simulink model "VCU_CS75_12_27_test"  (R2014a)
settings: Solver=FixedStepDiscrete  StartTime=0.0  StopTime=25  FixedStep=0.0005  RelTol=1e-3
undefined symbols (not defined in the file): D1, D2, D3, ecucoder_acal, ErrorSumMax1, ErrorSumMax2, ErrorSumMax3, I1, I2, I3, I_SW01_L, LaterlAngleCommand, LDW, P1, P2, P3, RemoteAcclPosition
libraries: simulink x913, ec5744lib x39
(part 20 of 30)

== system VCU_CS75_12_27_test/长安CS75底盘程序，20ms一次/Output/Subsystem/TransmitMessages10/LAS_29D/LAS_VoiceWarning ==
  LAS_VoiceWarning : Inport
  Constant{1..2,4..8} (7 alike) : Constant  Value=0  OutDataTypeStr=uint8
  LAS_VoiceWarningRon : Rounding  Operator=round
  LAS_VoiceWarning_1sat : Saturate  UpperLimit=192  LowerLimit=0
  LAS_VoiceWarning_Convert : DataTypeConversion  OutDataTypeStr=uint8
  LAS_VoiceWarning_Convert1 : DataTypeConversion  OutDataTypeStr=uint32
  LAS_VoiceWarning_D : Product  Inputs=*/
  LAS_VoiceWarning_F : Constant  OutDataTypeStr=single
  LAS_VoiceWarning_L : simulink/Logic and Bit Operations/Bitwise Operator  logicop=AND  UseBitMask=on  BitMask=192  BitMaskRealWorld=Stored Integer
  LAS_VoiceWarning_O : Constant  Value=0  OutDataTypeStr=single
  LAS_VoiceWarning_S : ArithShift  BitShiftNumber=-6
  LAS_VoiceWarning_sat : Saturate  UpperLimit=0  LowerLimit=0
  LAS_VoiceWarning_st : Sum  Inputs=+-
  output1 : Outport
  output2 : Outport  Port=2
  output3 : Outport  Port=3
  output4 : Outport  Port=4
  output5 : Outport  Port=5
  output6 : Outport  Port=6
  output7 : Outport  Port=7
  output8 : Outport  Port=8
  wires:
  LAS_VoiceWarning/1 -> LAS_VoiceWarning_sat/1
  LAS_VoiceWarning_sat/1 -> LAS_VoiceWarning_st/1
  LAS_VoiceWarning_O/1 -> LAS_VoiceWarning_st/2
  LAS_VoiceWarning_st/1 -> LAS_VoiceWarning_D/1
  LAS_VoiceWarning_F/1 -> LAS_VoiceWarning_D/2
  LAS_VoiceWarning_D/1 -> LAS_VoiceWarningRon/1
  LAS_VoiceWarningRon/1 -> LAS_VoiceWarning_S/1
  LAS_VoiceWarning_S/1 -> LAS_VoiceWarning_1sat/1
  LAS_VoiceWarning_1sat/1 -> LAS_VoiceWarning_Convert1/1
  LAS_VoiceWarning_Convert1/1 -> LAS_VoiceWarning_L/1
  LAS_VoiceWarning_L/1 -> LAS_VoiceWarning_Convert/1
  LAS_VoiceWarning_Convert/1 -> output3/1
  Constant1/1 -> output1/1
  Constant2/1 -> output2/1
  Constant4/1 -> output4/1
  Constant5/1 -> output5/1
  Constant6/1 -> output6/1
  Constant7/1 -> output7/1
  Constant8/1 -> output8/1

== system VCU_CS75_12_27_test/长安CS75底盘程序，20ms一次/Output/Subsystem/TransmitMessages10/LAS_29D/RollingConter ==
  RollingConter : Inport
  Constant{1..6,8} (7 alike) : Constant  Value=0  OutDataTypeStr=uint8
  RollingConterRon : Rounding  Operator=round
  RollingConter_1sat : Saturate  UpperLimit=15  LowerLimit=0
  RollingConter_Convert : DataTypeConversion  OutDataTypeStr=uint8
  RollingConter_Convert1 : DataTypeConversion  OutDataTypeStr=uint32
  RollingConter_D : Product  Inputs=*/
  RollingConter_F : Constant  OutDataTypeStr=single
  RollingConter_L : simulink/Logic and Bit Operations/Bitwise Operator  logicop=AND  UseBitMask=on  BitMask=15  BitMaskRealWorld=Stored Integer
  RollingConter_O : Constant  Value=0  OutDataTypeStr=single
  RollingConter_S : ArithShift
  RollingConter_sat : Saturate  UpperLimit=0  LowerLimit=0
  RollingConter_st : Sum  Inputs=+-
  output1 : Outport
  output2 : Outport  Port=2
  output3 : Outport  Port=3
  output4 : Outport  Port=4
  output5 : Outport  Port=5
  output6 : Outport  Port=6
  output7 : Outport  Port=7
  output8 : Outport  Port=8
  wires:
  RollingConter/1 -> RollingConter_sat/1
  RollingConter_sat/1 -> RollingConter_st/1
  RollingConter_O/1 -> RollingConter_st/2
  RollingConter_st/1 -> RollingConter_D/1
  RollingConter_F/1 -> RollingConter_D/2
  RollingConter_D/1 -> RollingConterRon/1
  RollingConterRon/1 -> RollingConter_S/1
  RollingConter_S/1 -> RollingConter_1sat/1
  RollingConter_1sat/1 -> RollingConter_Convert1/1
  RollingConter_Convert1/1 -> RollingConter_L/1
  RollingConter_L/1 -> RollingConter_Convert/1
  RollingConter_Convert/1 -> output7/1
  Constant1/1 -> output1/1
  Constant2/1 -> output2/1
  Constant3/1 -> output3/1
  Constant4/1 -> output4/1
  Constant5/1 -> output5/1
  Constant6/1 -> output6/1
  Constant8/1 -> output8/1

== system VCU_CS75_12_27_test/长安CS75底盘程序，20ms一次/Output/Subsystem/TransmitMessages11/GW_LCDAL_2EA/LCDAL_AudioWarningEnableStatus ==
  LCDAL_AudioWarningEnableStatus : Inport
  Constant{1..4,6..8} (7 alike) : Constant  Value=0  OutDataTypeStr=uint8
  LCDAL_AudioWarningEnableStatusABS : Abs
  LCDAL_AudioWarningEnableStatusCS : ArithShift  BitShiftNumber=-2
  LCDAL_AudioWarningEnableStatusConS : Constant  OutDataTypeStr=single
  LCDAL_AudioWarningEnableStatusCosR : Constant  Value=0  OutDataTypeStr=uint8
  LCDAL_AudioWarningEnableStatusROP : RelationalOperator  Operator=<  OutDataTypeStr=boolean
  LCDAL_AudioWarningEnableStatusRon : Rounding  Operator=round
  LCDAL_AudioWarningEnableStatusSW : Switch  Criteria=u2 ~= 0
  LCDAL_AudioWarningEnableStatus_1sat : Saturate  UpperLimit=192  LowerLimit=0
  LCDAL_AudioWarningEnableStatus_Convert : DataTypeConversion  OutDataTypeStr=uint8
  LCDAL_AudioWarningEnableStatus_Convert1 : DataTypeConversion  OutDataTypeStr=uint32
  LCDAL_AudioWarningEnableStatus_D : Product  Inputs=*/
  LCDAL_AudioWarningEnableStatus_F : Constant  OutDataTypeStr=single
  LCDAL_AudioWarningEnableStatus_L : simulink/Logic and Bit Operations/Bitwise Operator  logicop=AND  UseBitMask=on  BitMask=192  BitMaskRealWorld=Stored Integer
  LCDAL_AudioWarningEnableStatus_O : Constant  Value=0  OutDataTypeStr=single
  LCDAL_AudioWarningEnableStatus_S : ArithShift  BitShiftNumber=-6
  LCDAL_AudioWarningEnableStatus_sat : Saturate  UpperLimit=3  LowerLimit=0
  LCDAL_AudioWarningEnableStatus_st : Sum  Inputs=+-
  LCDAL_AudioWarningEnableStatussubcon : Sum  Inputs=+-
  output1 : Outport
  output2 : Outport  Port=2
  output3 : Outport  Port=3
  output4 : Outport  Port=4
  output5 : Outport  Port=5
  output6 : Outport  Port=6
  output7 : Outport  Port=7
  output8 : Outport  Port=8
  wires:
  Constant8/1 -> output8/1
  Constant7/1 -> output7/1
  Constant6/1 -> output6/1
  Constant4/1 -> output4/1
  Constant3/1 -> output3/1
  Constant2/1 -> output2/1
  Constant1/1 -> output1/1
  LCDAL_AudioWarningEnableStatus_Convert/1 -> output5/1
  LCDAL_AudioWarningEnableStatus_L/1 -> LCDAL_AudioWarningEnableStatus_Convert/1
  LCDAL_AudioWarningEnableStatus_Convert1/1 -> LCDAL_AudioWarningEnableStatus_L/1
  LCDAL_AudioWarningEnableStatus_1sat/1 -> LCDAL_AudioWarningEnableStatus_Convert1/1
  LCDAL_AudioWarningEnableStatus_S/1 -> LCDAL_AudioWarningEnableStatus_1sat/1
  LCDAL_AudioWarningEnableStatusSW/1 -> LCDAL_AudioWarningEnableStatus_S/1
  LCDAL_AudioWarningEnableStatusROP/1 -> LCDAL_AudioWarningEnableStatusSW/2
  LCDAL_AudioWarningEnableStatussubcon/1 -> LCDAL_AudioWarningEnableStatusSW/1
  LCDAL_AudioWarningEnableStatusABS/1 -> LCDAL_AudioWarningEnableStatussubcon/2
  LCDAL_AudioWarningEnableStatusCS/1 -> LCDAL_AudioWarningEnableStatussubcon/1
  LCDAL_AudioWarningEnableStatusConS/1 -> LCDAL_AudioWarningEnableStatusCS/1
  LCDAL_AudioWarningEnableStatusCosR/1 -> LCDAL_AudioWarningEnableStatusROP/2
  LCDAL_AudioWarningEnableStatusRon/1 -> LCDAL_AudioWarningEnableStatusSW/3, LCDAL_AudioWarningEnableStatusABS/1, LCDAL_AudioWarningEnableStatusROP/1
  LCDAL_AudioWarningEnableStatus_D/1 -> LCDAL_AudioWarningEnableStatusRon/1
  LCDAL_AudioWarningEnableStatus_F/1 -> LCDAL_AudioWarningEnableStatus_D/2
  LCDAL_AudioWarningEnableStatus_st/1 -> LCDAL_AudioWarningEnableStatus_D/1
  LCDAL_AudioWarningEnableStatus_O/1 -> LCDAL_AudioWarningEnableStatus_st/2
  LCDAL_AudioWarningEnableStatus_sat/1 -> LCDAL_AudioWarningEnableStatus_st/1
  LCDAL_AudioWarningEnableStatus/1 -> LCDAL_AudioWarningEnableStatus_sat/1

== system VCU_CS75_12_27_test/长安CS75底盘程序，20ms一次/Output/Subsystem/TransmitMessages11/GW_LCDAL_2EA/LCDAL_BSDLCAAlert ==
  LCDAL_BSDLCAAlert : Inport
  Constant{2..8} (7 alike) : Constant  Value=0  OutDataTypeStr=uint8
  LCDAL_BSDLCAAlertRon : Rounding  Operator=round
  LCDAL_BSDLCAAlert_1sat : Saturate  UpperLimit=48  LowerLimit=0
  LCDAL_BSDLCAAlert_Convert : DataTypeConversion  OutDataTypeStr=uint8
  LCDAL_BSDLCAAlert_Convert1 : DataTypeConversion  OutDataTypeStr=uint32
  LCDAL_BSDLCAAlert_D : Product  Inputs=*/
  LCDAL_BSDLCAAlert_F : Constant  OutDataTypeStr=single
  LCDAL_BSDLCAAlert_L : simulink/Logic and Bit Operations/Bitwise Operator  logicop=AND  UseBitMask=on  BitMask=48  BitMaskRealWorld=Stored Integer
  LCDAL_BSDLCAAlert_O : Constant  Value=0  OutDataTypeStr=single
  LCDAL_BSDLCAAlert_S : ArithShift  BitShiftNumber=-4
  LCDAL_BSDLCAAlert_sat : Saturate  UpperLimit=3  LowerLimit=0
  LCDAL_BSDLCAAlert_st : Sum  Inputs=+-
  output1 : Outport
  output2 : Outport  Port=2
  output3 : Outport  Port=3
  output4 : Outport  Port=4
  output5 : Outport  Port=5
  output6 : Outport  Port=6
  output7 : Outport  Port=7
  output8 : Outport  Port=8
  wires:
  Constant8/1 -> output8/1
  Constant7/1 -> output7/1
  Constant6/1 -> output6/1
  Constant5/1 -> output5/1
  Constant4/1 -> output4/1
  Constant3/1 -> output3/1
  Constant2/1 -> output2/1
  LCDAL_BSDLCAAlert_Convert/1 -> output1/1
  LCDAL_BSDLCAAlert_L/1 -> LCDAL_BSDLCAAlert_Convert/1
  LCDAL_BSDLCAAlert_Convert1/1 -> LCDAL_BSDLCAAlert_L/1
  LCDAL_BSDLCAAlert_1sat/1 -> LCDAL_BSDLCAAlert_Convert1/1
  LCDAL_BSDLCAAlert_S/1 -> LCDAL_BSDLCAAlert_1sat/1
  LCDAL_BSDLCAAlertRon/1 -> LCDAL_BSDLCAAlert_S/1
  LCDAL_BSDLCAAlert_D/1 -> LCDAL_BSDLCAAlertRon/1
  LCDAL_BSDLCAAlert_F/1 -> LCDAL_BSDLCAAlert_D/2
  LCDAL_BSDLCAAlert_st/1 -> LCDAL_BSDLCAAlert_D/1
  LCDAL_BSDLCAAlert_O/1 -> LCDAL_BSDLCAAlert_st/2
  LCDAL_BSDLCAAlert_sat/1 -> LCDAL_BSDLCAAlert_st/1
  LCDAL_BSDLCAAlert/1 -> LCDAL_BSDLCAAlert_sat/1

== system VCU_CS75_12_27_test/长安CS75底盘程序，20ms一次/Output/Subsystem/TransmitMessages11/GW_LCDAL_2EA/LCDAL_BSDLCAEnableStatus ==
  LCDAL_BSDLCAEnableStatus : Inport
  Constant{2..8} (7 alike) : Constant  Value=0  OutDataTypeStr=uint8
  LCDAL_BSDLCAEnableStatusRon : Rounding  Operator=round
  LCDAL_BSDLCAEnableStatus_1sat : Saturate  UpperLimit=192  LowerLimit=0
  LCDAL_BSDLCAEnableStatus_Convert : DataTypeConversion  OutDataTypeStr=uint8
  LCDAL_BSDLCAEnableStatus_Convert1 : DataTypeConversion  OutDataTypeStr=uint32
  LCDAL_BSDLCAEnableStatus_D : Product  Inputs=*/
  LCDAL_BSDLCAEnableStatus_F : Constant  OutDataTypeStr=single
  LCDAL_BSDLCAEnableStatus_L : simulink/Logic and Bit Operations/Bitwise Operator  logicop=AND  UseBitMask=on  BitMask=192  BitMaskRealWorld=Stored Integer
  LCDAL_BSDLCAEnableStatus_O : Constant  Value=0  OutDataTypeStr=single
  LCDAL_BSDLCAEnableStatus_S : ArithShift  BitShiftNumber=-6
  LCDAL_BSDLCAEnableStatus_sat : Saturate  UpperLimit=3  LowerLimit=0
  LCDAL_BSDLCAEnableStatus_st : Sum  Inputs=+-
  output1 : Outport
  output2 : Outport  Port=2
  output3 : Outport  Port=3
  output4 : Outport  Port=4
  output5 : Outport  Port=5
  output6 : Outport  Port=6
  output7 : Outport  Port=7
  output8 : Outport  Port=8
  wires:
  Constant8/1 -> output8/1
  Constant7/1 -> output7/1
  Constant6/1 -> output6/1
  Constant5/1 -> output5/1
  Constant4/1 -> output4/1
  Constant3/1 -> output3/1
  Constant2/1 -> output2/1
  LCDAL_BSDLCAEnableStatus_Convert/1 -> output1/1
  LCDAL_BSDLCAEnableStatus_L/1 -> LCDAL_BSDLCAEnableStatus_Convert/1
  LCDAL_BSDLCAEnableStatus_Convert1/1 -> LCDAL_BSDLCAEnableStatus_L/1
  LCDAL_BSDLCAEnableStatus_1sat/1 -> LCDAL_BSDLCAEnableStatus_Convert1/1
  LCDAL_BSDLCAEnableStatus_S/1 -> LCDAL_BSDLCAEnableStatus_1sat/1
  LCDAL_BSDLCAEnableStatusRon/1 -> LCDAL_BSDLCAEnableStatus_S/1
  LCDAL_BSDLCAEnableStatus_D/1 -> LCDAL_BSDLCAEnableStatusRon/1
  LCDAL_BSDLCAEnableStatus_F/1 -> LCDAL_BSDLCAEnableStatus_D/2
  LCDAL_BSDLCAEnableStatus_st/1 -> LCDAL_BSDLCAEnableStatus_D/1
  LCDAL_BSDLCAEnableStatus_O/1 -> LCDAL_BSDLCAEnableStatus_st/2
  LCDAL_BSDLCAEnableStatus_sat/1 -> LCDAL_BSDLCAEnableStatus_st/1
  LCDAL_BSDLCAEnableStatus/1 -> LCDAL_BSDLCAEnableStatus_sat/1

== system VCU_CS75_12_27_test/长安CS75底盘程序，20ms一次/Output/Subsystem/TransmitMessages11/GW_LCDAL_2EA/LCDAL_BSDLCAStatus ==
  LCDAL_BSDLCAStatus : Inport
  Constant{1,3..8} (7 alike) : Constant  Value=0  OutDataTypeStr=uint8
  LCDAL_BSDLCAStatusRon : Rounding  Operator=round
  LCDAL_BSDLCAStatus_1sat : Saturate  UpperLimit=24  LowerLimit=0
  LCDAL_BSDLCAStatus_Convert : DataTypeConversion  OutDataTypeStr=uint8
  LCDAL_BSDLCAStatus_Convert1 : DataTypeConversion  OutDataTypeStr=uint32
  LCDAL_BSDLCAStatus_D : Product  Inputs=*/
  LCDAL_BSDLCAStatus_F : Constant  OutDataTypeStr=single
  LCDAL_BSDLCAStatus_L : simulink/Logic and Bit Operations/Bitwise Operator  logicop=AND  UseBitMask=on  BitMask=24  BitMaskRealWorld=Stored Integer
  LCDAL_BSDLCAStatus_O : Constant  Value=0  OutDataTypeStr=single
  LCDAL_BSDLCAStatus_S : ArithShift  BitShiftNumber=-3
  LCDAL_BSDLCAStatus_sat : Saturate  UpperLimit=3  LowerLimit=0
  LCDAL_BSDLCAStatus_st : Sum  Inputs=+-
  output1 : Outport
  output2 : Outport  Port=2
  output3 : Outport  Port=3
  output4 : Outport  Port=4
  output5 : Outport  Port=5
  output6 : Outport  Port=6
  output7 : Outport  Port=7
  output8 : Outport  Port=8
  wires:
  Constant8/1 -> output8/1
  Constant7/1 -> output7/1
  Constant6/1 -> output6/1
  Constant5/1 -> output5/1
  Constant4/1 -> output4/1
  Constant3/1 -> output3/1
  Constant1/1 -> output1/1
  LCDAL_BSDLCAStatus_Convert/1 -> output2/1
  LCDAL_BSDLCAStatus_L/1 -> LCDAL_BSDLCAStatus_Convert/1
  LCDAL_BSDLCAStatus_Convert1/1 -> LCDAL_BSDLCAStatus_L/1
  LCDAL_BSDLCAStatus_1sat/1 -> LCDAL_BSDLCAStatus_Convert1/1
  LCDAL_BSDLCAStatus_S/1 -> LCDAL_BSDLCAStatus_1sat/1
  LCDAL_BSDLCAStatusRon/1 -> LCDAL_BSDLCAStatus_S/1
  LCDAL_BSDLCAStatus_D/1 -> LCDAL_BSDLCAStatusRon/1
  LCDAL_BSDLCAStatus_F/1 -> LCDAL_BSDLCAStatus_D/2
  LCDAL_BSDLCAStatus_st/1 -> LCDAL_BSDLCAStatus_D/1
  LCDAL_BSDLCAStatus_O/1 -> LCDAL_BSDLCAStatus_st/2
  LCDAL_BSDLCAStatus_sat/1 -> LCDAL_BSDLCAStatus_st/1
  LCDAL_BSDLCAStatus/1 -> LCDAL_BSDLCAStatus_sat/1

== system VCU_CS75_12_27_test/长安CS75底盘程序，20ms一次/Output/Subsystem/TransmitMessages11/GW_LCDAL_2EA/LCDAL_CTAAlert ==
  LCDAL_CTAAlert : Inport
  Constant{2..8} (7 alike) : Constant  Value=0  OutDataTypeStr=uint8
  LCDAL_CTAAlertABS : Abs
  LCDAL_CTAAlertCS : ArithShift  BitShiftNumber=-2
  LCDAL_CTAAlertConS : Constant  OutDataTypeStr=single
  LCDAL_CTAAlertCosR : Constant  Value=0  OutDataTypeStr=uint8
  LCDAL_CTAAlertROP : RelationalOperator  Operator=<  OutDataTypeStr=boolean
  LCDAL_CTAAlertRon : Rounding  Operator=round
  LCDAL_CTAAlertSW : Switch  Criteria=u2 ~= 0
  LCDAL_CTAAlert_1sat : Saturate  UpperLimit=3  LowerLimit=0
  LCDAL_CTAAlert_Convert : DataTypeConversion  OutDataTypeStr=uint8
  LCDAL_CTAAlert_Convert1 : DataTypeConversion  OutDataTypeStr=uint32
  LCDAL_CTAAlert_D : Product  Inputs=*/
  LCDAL_CTAAlert_F : Constant  OutDataTypeStr=single
  LCDAL_CTAAlert_L : simulink/Logic and Bit Operations/Bitwise Operator  logicop=AND  UseBitMask=on  BitMask=3  BitMaskRealWorld=Stored Integer
  LCDAL_CTAAlert_O : Constant  Value=0  OutDataTypeStr=single
  LCDAL_CTAAlert_S : ArithShift
  LCDAL_CTAAlert_sat : Saturate  UpperLimit=3  LowerLimit=0
  LCDAL_CTAAlert_st : Sum  Inputs=+-
  LCDAL_CTAAlertsubcon : Sum  Inputs=+-
  output1 : Outport
  output2 : Outport  Port=2
  output3 : Outport  Port=3
  output4 : Outport  Port=4
  output5 : Outport  Port=5
  output6 : Outport  Port=6
  output7 : Outport  Port=7
  output8 : Outport  Port=8
  wires:
  Constant8/1 -> output8/1
  Constant7/1 -> output7/1
  Constant6/1 -> output6/1
  Constant5/1 -> output5/1
  Constant4/1 -> output4/1
  Constant3/1 -> output3/1
  Constant2/1 -> output2/1
  LCDAL_CTAAlert_Convert/1 -> output1/1
  LCDAL_CTAAlert_L/1 -> LCDAL_CTAAlert_Convert/1
  LCDAL_CTAAlert_Convert1/1 -> LCDAL_CTAAlert_L/1
  LCDAL_CTAAlert_1sat/1 -> LCDAL_CTAAlert_Convert1/1
  LCDAL_CTAAlert_S/1 -> LCDAL_CTAAlert_1sat/1
  LCDAL_CTAAlertSW/1 -> LCDAL_CTAAlert_S/1
  LCDAL_CTAAlertROP/1 -> LCDAL_CTAAlertSW/2
  LCDAL_CTAAlertsubcon/1 -> LCDAL_CTAAlertSW/1
  LCDAL_CTAAlertABS/1 -> LCDAL_CTAAlertsubcon/2
  LCDAL_CTAAlertCS/1 -> LCDAL_CTAAlertsubcon/1
  LCDAL_CTAAlertConS/1 -> LCDAL_CTAAlertCS/1
  LCDAL_CTAAlertCosR/1 -> LCDAL_CTAAlertROP/2
  LCDAL_CTAAlertRon/1 -> LCDAL_CTAAlertSW/3, LCDAL_CTAAlertABS/1, LCDAL_CTAAlertROP/1
  LCDAL_CTAAlert_D/1 -> LCDAL_CTAAlertRon/1
  LCDAL_CTAAlert_F/1 -> LCDAL_CTAAlert_D/2
  LCDAL_CTAAlert_st/1 -> LCDAL_CTAAlert_D/1
  LCDAL_CTAAlert_O/1 -> LCDAL_CTAAlert_st/2
  LCDAL_CTAAlert_sat/1 -> LCDAL_CTAAlert_st/1
  LCDAL_CTAAlert/1 -> LCDAL_CTAAlert_sat/1

== system VCU_CS75_12_27_test/长安CS75底盘程序，20ms一次/Output/Subsystem/TransmitMessages11/GW_LCDAL_2EA/LCDAL_CTAEnableStatus ==
  LCDAL_CTAEnableStatus : Inport
  Constant{1..3,5..8} (7 alike) : Constant  Value=0  OutDataTypeStr=uint8
  LCDAL_CTAEnableStatusRon : Rounding  Operator=round
  LCDAL_CTAEnableStatus_1sat : Saturate  UpperLimit=192  LowerLimit=0
  LCDAL_CTAEnableStatus_Convert : DataTypeConversion  OutDataTypeStr=uint8
  LCDAL_CTAEnableStatus_Convert1 : DataTypeConversion  OutDataTypeStr=uint32
  LCDAL_CTAEnableStatus_D : Product  Inputs=*/
  LCDAL_CTAEnableStatus_F : Constant  OutDataTypeStr=single
  LCDAL_CTAEnableStatus_L : simulink/Logic and Bit Operations/Bitwise Operator  logicop=AND  UseBitMask=on  BitMask=192  BitMaskRealWorld=Stored Integer
  LCDAL_CTAEnableStatus_O : Constant  Value=0  OutDataTypeStr=single
  LCDAL_CTAEnableStatus_S : ArithShift  BitShiftNumber=-6
  LCDAL_CTAEnableStatus_sat : Saturate  UpperLimit=3  LowerLimit=0
  LCDAL_CTAEnableStatus_st : Sum  Inputs=+-
  output1 : Outport
  output2 : Outport  Port=2
  output3 : Outport  Port=3
  output4 : Outport  Port=4
  output5 : Outport  Port=5
  output6 : Outport  Port=6
  output7 : Outport  Port=7
  output8 : Outport  Port=8
  wires:
  Constant8/1 -> output8/1
  Constant7/1 -> output7/1
  Constant6/1 -> output6/1
  Constant5/1 -> output5/1
  Constant3/1 -> output3/1
  Constant2/1 -> output2/1
  Constant1/1 -> output1/1
  LCDAL_CTAEnableStatus_Convert/1 -> output4/1
  LCDAL_CTAEnableStatus_L/1 -> LCDAL_CTAEnableStatus_Convert/1
  LCDAL_CTAEnableStatus_Convert1/1 -> LCDAL_CTAEnableStatus_L/1
  LCDAL_CTAEnableStatus_1sat/1 -> LCDAL_CTAEnableStatus_Convert1/1
  LCDAL_CTAEnableStatus_S/1 -> LCDAL_CTAEnableStatus_1sat/1
  LCDAL_CTAEnableStatusRon/1 -> LCDAL_CTAEnableStatus_S/1
  LCDAL_CTAEnableStatus_D/1 -> LCDAL_CTAEnableStatusRon/1
  LCDAL_CTAEnableStatus_F/1 -> LCDAL_CTAEnableStatus_D/2
  LCDAL_CTAEnableStatus_st/1 -> LCDAL_CTAEnableStatus_D/1
  LCDAL_CTAEnableStatus_O/1 -> LCDAL_CTAEnableStatus_st/2
  LCDAL_CTAEnableStatus_sat/1 -> LCDAL_CTAEnableStatus_st/1
  LCDAL_CTAEnableStatus/1 -> LCDAL_CTAEnableStatus_sat/1

== system VCU_CS75_12_27_test/长安CS75底盘程序，20ms一次/Output/Subsystem/TransmitMessages11/GW_LCDAL_2EA/LCDAL_CTAStatus ==
  LCDAL_CTAStatus : Inport
  Constant{1,3..8} (7 alike) : Constant  Value=0  OutDataTypeStr=uint8
  LCDAL_CTAStatusRon : Rounding  Operator=round
  LCDAL_CTAStatus_1sat : Saturate  UpperLimit=6  LowerLimit=0
  LCDAL_CTAStatus_Convert : DataTypeConversion  OutDataTypeStr=uint8
  LCDAL_CTAStatus_Convert1 : DataTypeConversion  OutDataTypeStr=uint32
  LCDAL_CTAStatus_D : Product  Inputs=*/
  LCDAL_CTAStatus_F : Constant  OutDataTypeStr=single
  LCDAL_CTAStatus_L : simulink/Logic and Bit Operations/Bitwise Operator  logicop=AND  UseBitMask=on  BitMask=6  BitMaskRealWorld=Stored Integer
  LCDAL_CTAStatus_O : Constant  Value=0  OutDataTypeStr=single
  LCDAL_CTAStatus_S : ArithShift  BitShiftNumber=-1
  LCDAL_CTAStatus_sat : Saturate  UpperLimit=3  LowerLimit=0
  LCDAL_CTAStatus_st : Sum  Inputs=+-
  output1 : Outport
  output2 : Outport  Port=2
  output3 : Outport  Port=3
  output4 : Outport  Port=4
  output5 : Outport  Port=5
  output6 : Outport  Port=6
  output7 : Outport  Port=7
  output8 : Outport  Port=8
  wires:
  Constant8/1 -> output8/1
  Constant7/1 -> output7/1
  Constant6/1 -> output6/1
  Constant5/1 -> output5/1
  Constant4/1 -> output4/1
  Constant3/1 -> output3/1
  Constant1/1 -> output1/1
  LCDAL_CTAStatus_Convert/1 -> output2/1
  LCDAL_CTAStatus_L/1 -> LCDAL_CTAStatus_Convert/1
  LCDAL_CTAStatus_Convert1/1 -> LCDAL_CTAStatus_L/1
  LCDAL_CTAStatus_1sat/1 -> LCDAL_CTAStatus_Convert1/1
  LCDAL_CTAStatus_S/1 -> LCDAL_CTAStatus_1sat/1
  LCDAL_CTAStatusRon/1 -> LCDAL_CTAStatus_S/1
  LCDAL_CTAStatus_D/1 -> LCDAL_CTAStatusRon/1
  LCDAL_CTAStatus_F/1 -> LCDAL_CTAStatus_D/2
  LCDAL_CTAStatus_st/1 -> LCDAL_CTAStatus_D/1
  LCDAL_CTAStatus_O/1 -> LCDAL_CTAStatus_st/2
  LCDAL_CTAStatus_sat/1 -> LCDAL_CTAStatus_st/1
  LCDAL_CTAStatus/1 -> LCDAL_CTAStatus_sat/1

== system VCU_CS75_12_27_test/长安CS75底盘程序，20ms一次/Output/Subsystem/TransmitMessages11/GW_LCDAL_2EA/LCDAL_LCATTCSettingStatus ==
  LCDAL_LCATTCSettingStatus : Inport
  Constant{1..4,6..8} (7 alike) : Constant  Value=0  OutDataTypeStr=uint8
  LCDAL_LCATTCSettingStatusABS : Abs
  LCDAL_LCATTCSettingStatusCS : ArithShift  BitShiftNumber=-2
  LCDAL_LCATTCSettingStatusConS : Constant  OutDataTypeStr=single
  LCDAL_LCATTCSettingStatusCosR : Constant  Value=0  OutDataTypeStr=uint8
  LCDAL_LCATTCSettingStatusROP : RelationalOperator  Operator=<  OutDataTypeStr=boolean
  LCDAL_LCATTCSettingStatusRon : Rounding  Operator=round
  LCDAL_LCATTCSettingStatusSW : Switch  Criteria=u2 ~= 0
  LCDAL_LCATTCSettingStatus_1sat : Saturate  UpperLimit=12  LowerLimit=0
  LCDAL_LCATTCSettingStatus_Convert : DataTypeConversion  OutDataTypeStr=uint8
  LCDAL_LCATTCSettingStatus_Convert1 : DataTypeConversion  OutDataTypeStr=uint32
  LCDAL_LCATTCSettingStatus_D : Product  Inputs=*/
  LCDAL_LCATTCSettingStatus_F : Constant  OutDataTypeStr=single
  LCDAL_LCATTCSettingStatus_L : simulink/Logic and Bit Operations/Bitwise Operator  logicop=AND  UseBitMask=on  BitMask=12  BitMaskRealWorld=Stored Integer
  LCDAL_LCATTCSettingStatus_O : Constant  Value=0  OutDataTypeStr=single
  LCDAL_LCATTCSettingStatus_S : ArithShift  BitShiftNumber=-2
  LCDAL_LCATTCSettingStatus_sat : Saturate  UpperLimit=3  LowerLimit=0
  LCDAL_LCATTCSettingStatus_st : Sum  Inputs=+-
  LCDAL_LCATTCSettingStatussubcon : Sum  Inputs=+-
  output1 : Outport
  output2 : Outport  Port=2
  output3 : Outport  Port=3
  output4 : Outport  Port=4
  output5 : Outport  Port=5
  output6 : Outport  Port=6
  output7 : Outport  Port=7
  output8 : Outport  Port=8
  wires:
  Constant8/1 -> output8/1
  Constant7/1 -> output7/1
  Constant6/1 -> output6/1
  Constant4/1 -> output4/1
  Constant3/1 -> output3/1
  Constant2/1 -> output2/1
  Constant1/1 -> output1/1
  LCDAL_LCATTCSettingStatus_Convert/1 -> output5/1
  LCDAL_LCATTCSettingStatus_L/1 -> LCDAL_LCATTCSettingStatus_Convert/1
  LCDAL_LCATTCSettingStatus_Convert1/1 -> LCDAL_LCATTCSettingStatus_L/1
  LCDAL_LCATTCSettingStatus_1sat/1 -> LCDAL_LCATTCSettingStatus_Convert1/1
  LCDAL_LCATTCSettingStatus_S/1 -> LCDAL_LCATTCSettingStatus_1sat/1
  LCDAL_LCATTCSettingStatusSW/1 -> LCDAL_LCATTCSettingStatus_S/1
  LCDAL_LCATTCSettingStatusROP/1 -> LCDAL_LCATTCSettingStatusSW/2
  LCDAL_LCATTCSettingStatussubcon/1 -> LCDAL_LCATTCSettingStatusSW/1
  LCDAL_LCATTCSettingStatusABS/1 -> LCDAL_LCATTCSettingStatussubcon/2
  LCDAL_LCATTCSettingStatusCS/1 -> LCDAL_LCATTCSettingStatussubcon/1
  LCDAL_LCATTCSettingStatusConS/1 -> LCDAL_LCATTCSettingStatusCS/1
  LCDAL_LCATTCSettingStatusCosR/1 -> LCDAL_LCATTCSettingStatusROP/2
  LCDAL_LCATTCSettingStatusRon/1 -> LCDAL_LCATTCSettingStatusSW/3, LCDAL_LCATTCSettingStatusABS/1, LCDAL_LCATTCSettingStatusROP/1
  LCDAL_LCATTCSettingStatus_D/1 -> LCDAL_LCATTCSettingStatusRon/1
  LCDAL_LCATTCSettingStatus_F/1 -> LCDAL_LCATTCSettingStatus_D/2
  LCDAL_LCATTCSettingStatus_st/1 -> LCDAL_LCATTCSettingStatus_D/1
  LCDAL_LCATTCSettingStatus_O/1 -> LCDAL_LCATTCSettingStatus_st/2
  LCDAL_LCATTCSettingStatus_sat/1 -> LCDAL_LCATTCSettingStatus_st/1
  LCDAL_LCATTCSettingStatus/1 -> LCDAL_LCATTCSettingStatus_sat/1

== system VCU_CS75_12_27_test/长安CS75底盘程序，20ms一次/Output/Subsystem/TransmitMessages11/GW_LCDAL_2EA/LCDAL_LockCtrlEnableStatus ==
  LCDAL_LockCtrlEnableStatus : Inport
  Constant{1..4,6..8} (7 alike) : Constant  Value=0  OutDataTypeStr=uint8
  LCDAL_LockCtrlEnableStatusABS : Abs
  LCDAL_LockCtrlEnableStatusCS : ArithShift  BitShiftNumber=-2
  LCDAL_LockCtrlEnableStatusConS : Constant  OutDataTypeStr=single
  LCDAL_LockCtrlEnableStatusCosR : Constant  Value=0  OutDataTypeStr=uint8
  LCDAL_LockCtrlEnableStatusROP : RelationalOperator  Operator=<  OutDataTypeStr=boolean
  LCDAL_LockCtrlEnableStatusRon : Rounding  Operator=round
  LCDAL_LockCtrlEnableStatusSW : Switch  Criteria=u2 ~= 0
  LCDAL_LockCtrlEnableStatus_1sat : Saturate  UpperLimit=48  LowerLimit=0
  LCDAL_LockCtrlEnableStatus_Convert : DataTypeConversion  OutDataTypeStr=uint8
  LCDAL_LockCtrlEnableStatus_Convert1 : DataTypeConversion  OutDataTypeStr=uint32
  LCDAL_LockCtrlEnableStatus_D : Product  Inputs=*/
  LCDAL_LockCtrlEnableStatus_F : Constant  OutDataTypeStr=single
  LCDAL_LockCtrlEnableStatus_L : simulink/Logic and Bit Operations/Bitwise Operator  logicop=AND  UseBitMask=on  BitMask=48  BitMaskRealWorld=Stored Integer
  LCDAL_LockCtrlEnableStatus_O : Constant  Value=0  OutDataTypeStr=single
  LCDAL_LockCtrlEnableStatus_S : ArithShift  BitShiftNumber=-4
  LCDAL_LockCtrlEnableStatus_sat : Saturate  UpperLimit=3  LowerLimit=0
  LCDAL_LockCtrlEnableStatus_st : Sum  Inputs=+-
  LCDAL_LockCtrlEnableStatussubcon : Sum  Inputs=+-
  output1 : Outport
  output2 : Outport  Port=2
  output3 : Outport  Port=3
  output4 : Outport  Port=4
  output5 : Outport  Port=5
  output6 : Outport  Port=6
  output7 : Outport  Port=7
  output8 : Outport  Port=8
  wires:
  Constant8/1 -> output8/1
  Constant7/1 -> output7/1
  Constant6/1 -> output6/1
  Constant4/1 -> output4/1
  Constant3/1 -> output3/1
  Constant2/1 -> output2/1
  Constant1/1 -> output1/1
  LCDAL_LockCtrlEnableStatus_Convert/1 -> output5/1
  LCDAL_LockCtrlEnableStatus_L/1 -> LCDAL_LockCtrlEnableStatus_Convert/1
  LCDAL_LockCtrlEnableStatus_Convert1/1 -> LCDAL_LockCtrlEnableStatus_L/1
  LCDAL_LockCtrlEnableStatus_1sat/1 -> LCDAL_LockCtrlEnableStatus_Convert1/1
  LCDAL_LockCtrlEnableStatus_S/1 -> LCDAL_LockCtrlEnableStatus_1sat/1
  LCDAL_LockCtrlEnableStatusSW/1 -> LCDAL_LockCtrlEnableStatus_S/1
  LCDAL_LockCtrlEnableStatusROP/1 -> LCDAL_LockCtrlEnableStatusSW/2
  LCDAL_LockCtrlEnableStatussubcon/1 -> LCDAL_LockCtrlEnableStatusSW/1
  LCDAL_LockCtrlEnableStatusABS/1 -> LCDAL_LockCtrlEnableStatussubcon/2
  LCDAL_LockCtrlEnableStatusCS/1 -> LCDAL_LockCtrlEnableStatussubcon/1
  LCDAL_LockCtrlEnableStatusConS/1 -> LCDAL_LockCtrlEnableStatusCS/1
  LCDAL_LockCtrlEnableStatusCosR/1 -> LCDAL_LockCtrlEnableStatusROP/2
  LCDAL_LockCtrlEnableStatusRon/1 -> LCDAL_LockCtrlEnableStatusSW/3, LCDAL_LockCtrlEnableStatusABS/1, LCDAL_LockCtrlEnableStatusROP/1
  LCDAL_LockCtrlEnableStatus_D/1 -> LCDAL_LockCtrlEnableStatusRon/1
  LCDAL_LockCtrlEnableStatus_F/1 -> LCDAL_LockCtrlEnableStatus_D/2
  LCDAL_LockCtrlEnableStatus_st/1 -> LCDAL_LockCtrlEnableStatus_D/1
  LCDAL_LockCtrlEnableStatus_O/1 -> LCDAL_LockCtrlEnableStatus_st/2
  LCDAL_LockCtrlEnableStatus_sat/1 -> LCDAL_LockCtrlEnableStatus_st/1
  LCDAL_LockCtrlEnableStatus/1 -> LCDAL_LockCtrlEnableStatus_sat/1

== system VCU_CS75_12_27_test/长安CS75底盘程序，20ms一次/Output/Subsystem/TransmitMessages11/GW_LCDAL_2EA/LCDAL_RCWAlert ==
  LCDAL_RCWAlert : Inport
  Constant{1..2,4..8} (7 alike) : Constant  Value=0  OutDataTypeStr=uint8
  LCDAL_RCWAlertRon : Rounding  Operator=round
  LCDAL_RCWAlert_1sat : Saturate  UpperLimit=3  LowerLimit=0
  LCDAL_RCWAlert_Convert : DataTypeConversion  OutDataTypeStr=uint8
  LCDAL_RCWAlert_Convert1 : DataTypeConversion  OutDataTypeStr=uint32
  LCDAL_RCWAlert_D : Product  Inputs=*/
  LCDAL_RCWAlert_F : Constant  OutDataTypeStr=single
  LCDAL_RCWAlert_L : simulink/Logic and Bit Operations/Bitwise Operator  logicop=AND  UseBitMask=on  BitMask=3  BitMaskRealWorld=Stored Integer
  LCDAL_RCWAlert_O : Constant  Value=0  OutDataTypeStr=single
  LCDAL_RCWAlert_S : ArithShift
  LCDAL_RCWAlert_sat : Saturate  UpperLimit=3  LowerLimit=0
  LCDAL_RCWAlert_st : Sum  Inputs=+-
  output1 : Outport
  output2 : Outport  Port=2
  output3 : Outport  Port=3
  output4 : Outport  Port=4
  output5 : Outport  Port=5
  output6 : Outport  Port=6
  output7 : Outport  Port=7
  output8 : Outport  Port=8
  wires:
  Constant8/1 -> output8/1
  Constant7/1 -> output7/1
  Constant6/1 -> output6/1
  Constant5/1 -> output5/1
  Constant4/1 -> output4/1
  Constant2/1 -> output2/1
  Constant1/1 -> output1/1
  LCDAL_RCWAlert_Convert/1 -> output3/1
  LCDAL_RCWAlert_L/1 -> LCDAL_RCWAlert_Convert/1
  LCDAL_RCWAlert_Convert1/1 -> LCDAL_RCWAlert_L/1
  LCDAL_RCWAlert_1sat/1 -> LCDAL_RCWAlert_Convert1/1
  LCDAL_RCWAlert_S/1 -> LCDAL_RCWAlert_1sat/1
  LCDAL_RCWAlertRon/1 -> LCDAL_RCWAlert_S/1
  LCDAL_RCWAlert_D/1 -> LCDAL_RCWAlertRon/1
  LCDAL_RCWAlert_F/1 -> LCDAL_RCWAlert_D/2
  LCDAL_RCWAlert_st/1 -> LCDAL_RCWAlert_D/1
  LCDAL_RCWAlert_O/1 -> LCDAL_RCWAlert_st/2
  LCDAL_RCWAlert_sat/1 -> LCDAL_RCWAlert_st/1
  LCDAL_RCWAlert/1 -> LCDAL_RCWAlert_sat/1

== system VCU_CS75_12_27_test/长安CS75底盘程序，20ms一次/Output/Subsystem/TransmitMessages11/GW_LCDAL_2EA/LCDAL_RCWEnableStatus ==
  LCDAL_RCWEnableStatus : Inport
  Constant{1..2,4..8} (7 alike) : Constant  Value=0  OutDataTypeStr=uint8
  LCDAL_RCWEnableStatusRon : Rounding  Operator=round
  LCDAL_RCWEnableStatus_1sat : Saturate  UpperLimit=48  LowerLimit=0
  LCDAL_RCWEnableStatus_Convert : DataTypeConversion  OutDataTypeStr=uint8
  LCDAL_RCWEnableStatus_Convert1 : DataTypeConversion  OutDataTypeStr=uint32
  LCDAL_RCWEnableStatus_D : Product  Inputs=*/
  LCDAL_RCWEnableStatus_F : Constant  OutDataTypeStr=single
  LCDAL_RCWEnableStatus_L : simulink/Logic and Bit Operations/Bitwise Operator  logicop=AND  UseBitMask=on  BitMask=48  BitMaskRealWorld=Stored Integer
  LCDAL_RCWEnableStatus_O : Constant  Value=0  OutDataTypeStr=single
  LCDAL_RCWEnableStatus_S : ArithShift  BitShiftNumber=-4
  LCDAL_RCWEnableStatus_sat : Saturate  UpperLimit=3  LowerLimit=0
  LCDAL_RCWEnableStatus_st : Sum  Inputs=+-
  output1 : Outport
  output2 : Outport  Port=2
  output3 : Outport  Port=3
  output4 : Outport  Port=4
  output5 : Outport  Port=5
  output6 : Outport  Port=6
  output7 : Outport  Port=7
  output8 : Outport  Port=8
  wires:
  Constant8/1 -> output8/1
  Constant7/1 -> output7/1
  Constant6/1 -> output6/1
  Constant5/1 -> output5/1
  Constant4/1 -> output4/1
  Constant2/1 -> output2/1
  Constant1/1 -> output1/1
  LCDAL_RCWEnableStatus_Convert/1 -> output3/1
  LCDAL_RCWEnableStatus_L/1 -> LCDAL_RCWEnableStatus_Convert/1
  LCDAL_RCWEnableStatus_Convert1/1 -> LCDAL_RCWEnableStatus_L/1
  LCDAL_RCWEnableStatus_1sat/1 -> LCDAL_RCWEnableStatus_Convert1/1
  LCDAL_RCWEnableStatus_S/1 -> LCDAL_RCWEnableStatus_1sat/1
  LCDAL_RCWEnableStatusRon/1 -> LCDAL_RCWEnableStatus_S/1
  LCDAL_RCWEnableStatus_D/1 -> LCDAL_RCWEnableStatusRon/1
  LCDAL_RCWEnableStatus_F/1 -> LCDAL_RCWEnableStatus_D/2
  LCDAL_RCWEnableStatus_st/1 -> LCDAL_RCWEnableStatus_D/1
  LCDAL_RCWEnableStatus_O/1 -> LCDAL_RCWEnableStatus_st/2
  LCDAL_RCWEnableStatus_sat/1 -> LCDAL_RCWEnableStatus_st/1
  LCDAL_RCWEnableStatus/1 -> LCDAL_RCWEnableStatus_sat/1

== system VCU_CS75_12_27_test/长安CS75底盘程序，20ms一次/Output/Subsystem/TransmitMessages11/GW_LCDAL_2EA/LCDAL_RCWSoundEnableStatus ==
  LCDAL_RCWSoundEnableStatus : Inport
  Constant{1..3,5..8} (7 alike) : Constant  Value=0  OutDataTypeStr=uint8
  LCDAL_RCWSoundEnableStatusRon : Rounding  Operator=round
  LCDAL_RCWSoundEnableStatus_1sat : Saturate  UpperLimit=3  LowerLimit=0
  LCDAL_RCWSoundEnableStatus_Convert : DataTypeConversion  OutDataTypeStr=uint8
  LCDAL_RCWSoundEnableStatus_Convert1 : DataTypeConversion  OutDataTypeStr=uint32
  LCDAL_RCWSoundEnableStatus_D : Product  Inputs=*/
  LCDAL_RCWSoundEnableStatus_F : Constant  OutDataTypeStr=single
  LCDAL_RCWSoundEnableStatus_L : simulink/Logic and Bit Operations/Bitwise Operator  logicop=AND  UseBitMask=on  BitMask=3  BitMaskRealWorld=Stored Integer
  LCDAL_RCWSoundEnableStatus_O : Constant  Value=0  OutDataTypeStr=single
  LCDAL_RCWSoundEnableStatus_S : ArithShift
  LCDAL_RCWSoundEnableStatus_sat : Saturate  UpperLimit=3  LowerLimit=0
  LCDAL_RCWSoundEnableStatus_st : Sum  Inputs=+-
  output1 : Outport
  output2 : Outport  Port=2
  output3 : Outport  Port=3
  output4 : Outport  Port=4
  output5 : Outport  Port=5
  output6 : Outport  Port=6
  output7 : Outport  Port=7
  output8 : Outport  Port=8
  wires:
  Constant8/1 -> output8/1
  Constant7/1 -> output7/1
  Constant6/1 -> output6/1
  Constant5/1 -> output5/1
  Constant3/1 -> output3/1
  Constant2/1 -> output2/1
  Constant1/1 -> output1/1
  LCDAL_RCWSoundEnableStatus_Convert/1 -> output4/1
  LCDAL_RCWSoundEnableStatus_L/1 -> LCDAL_RCWSoundEnableStatus_Convert/1
  LCDAL_RCWSoundEnableStatus_Convert1/1 -> LCDAL_RCWSoundEnableStatus_L/1
  LCDAL_RCWSoundEnableStatus_1sat/1 -> LCDAL_RCWSoundEnableStatus_Convert1/1
  LCDAL_RCWSoundEnableStatus_S/1 -> LCDAL_RCWSoundEnableStatus_1sat/1
  LCDAL_RCWSoundEnableStatusRon/1 -> LCDAL_RCWSoundEnableStatus_S/1
  LCDAL_RCWSoundEnableStatus_D/1 -> LCDAL_RCWSoundEnableStatusRon/1
  LCDAL_RCWSoundEnableStatus_F/1 -> LCDAL_RCWSoundEnableStatus_D/2
  LCDAL_RCWSoundEnableStatus_st/1 -> LCDAL_RCWSoundEnableStatus_D/1
  LCDAL_RCWSoundEnableStatus_O/1 -> LCDAL_RCWSoundEnableStatus_st/2
  LCDAL_RCWSoundEnableStatus_sat/1 -> LCDAL_RCWSoundEnableStatus_st/1
  LCDAL_RCWSoundEnableStatus/1 -> LCDAL_RCWSoundEnableStatus_sat/1

== system VCU_CS75_12_27_test/长安CS75底盘程序，20ms一次/Output/Subsystem/TransmitMessages11/GW_LCDAL_2EA/LCDAL_RCWStatus ==
  LCDAL_RCWStatus : Inport
  Constant{1..3,5..8} (7 alike) : Constant  Value=0  OutDataTypeStr=uint8
  LCDAL_RCWStatusRon : Rounding  Operator=round
  LCDAL_RCWStatus_1sat : Saturate  UpperLimit=48  LowerLimit=0
  LCDAL_RCWStatus_Convert : DataTypeConversion  OutDataTypeStr=uint8
  LCDAL_RCWStatus_Convert1 : DataTypeConversion  OutDataTypeStr=uint32
  LCDAL_RCWStatus_D : Product  Inputs=*/
  LCDAL_RCWStatus_F : Constant  OutDataTypeStr=single
  LCDAL_RCWStatus_L : simulink/Logic and Bit Operations/Bitwise Operator  logicop=AND  UseBitMask=on  BitMask=48  BitMaskRealWorld=Stored Integer
  LCDAL_RCWStatus_O : Constant  Value=0  OutDataTypeStr=single
  LCDAL_RCWStatus_S : ArithShift  BitShiftNumber=-4
  LCDAL_RCWStatus_sat : Saturate  UpperLimit=3  LowerLimit=0
  LCDAL_RCWStatus_st : Sum  Inputs=+-
  output1 : Outport
  output2 : Outport  Port=2
  output3 : Outport  Port=3
  output4 : Outport  Port=4
  output5 : Outport  Port=5
  output6 : Outport  Port=6
  output7 : Outport  Port=7
  output8 : Outport  Port=8
  wires:
  Constant8/1 -> output8/1
  Constant7/1 -> output7/1
  Constant6/1 -> output6/1
  Constant5/1 -> output5/1
  Constant3/1 -> output3/1
  Constant2/1 -> output2/1
  Constant1/1 -> output1/1
  LCDAL_RCWStatus_Convert/1 -> output4/1
  LCDAL_RCWStatus_L/1 -> LCDAL_RCWStatus_Convert/1
  LCDAL_RCWStatus_Convert1/1 -> LCDAL_RCWStatus_L/1
  LCDAL_RCWStatus_1sat/1 -> LCDAL_RCWStatus_Convert1/1
  LCDAL_RCWStatus_S/1 -> LCDAL_RCWStatus_1sat/1
  LCDAL_RCWStatusRon/1 -> LCDAL_RCWStatus_S/1
  LCDAL_RCWStatus_D/1 -> LCDAL_RCWStatusRon/1
  LCDAL_RCWStatus_F/1 -> LCDAL_RCWStatus_D/2
  LCDAL_RCWStatus_st/1 -> LCDAL_RCWStatus_D/1
  LCDAL_RCWStatus_O/1 -> LCDAL_RCWStatus_st/2
  LCDAL_RCWStatus_sat/1 -> LCDAL_RCWStatus_st/1
  LCDAL_RCWStatus/1 -> LCDAL_RCWStatus_sat/1

== system VCU_CS75_12_27_test/长安CS75底盘程序，20ms一次/Output/Subsystem/TransmitMessages11/GW_LCDAL_2EA/LCDAL_SEAAlert ==
  LCDAL_SEAAlert : Inport
  Constant{2..8} (7 alike) : Constant  Value=0  OutDataTypeStr=uint8
  LCDAL_SEAAlertRon : Rounding  Operator=round
  LCDAL_SEAAlert_1sat : Saturate  UpperLimit=12  LowerLimit=0
  LCDAL_SEAAlert_Convert : DataTypeConversion  OutDataTypeStr=uint8
  LCDAL_SEAAlert_Convert1 : DataTypeConversion  OutDataTypeStr=uint32
  LCDAL_SEAAlert_D : Product  Inputs=*/
  LCDAL_SEAAlert_F : Constant  OutDataTypeStr=single
  LCDAL_SEAAlert_L : simulink/Logic and Bit Operations/Bitwise Operator  logicop=AND  UseBitMask=on  BitMask=12  BitMaskRealWorld=Stored Integer
  LCDAL_SEAAlert_O : Constant  Value=0  OutDataTypeStr=single
  LCDAL_SEAAlert_S : ArithShift  BitShiftNumber=-2
  LCDAL_SEAAlert_sat : Saturate  UpperLimit=3  LowerLimit=0
  LCDAL_SEAAlert_st : Sum  Inputs=+-
  output1 : Outport
  output2 : Outport  Port=2
  output3 : Outport  Port=3
  output4 : Outport  Port=4
  output5 : Outport  Port=5
  output6 : Outport  Port=6
  output7 : Outport  Port=7
  output8 : Outport  Port=8
  wires:
  Constant8/1 -> output8/1
  Constant7/1 -> output7/1
  Constant6/1 -> output6/1
  Constant5/1 -> output5/1
  Constant4/1 -> output4/1
  Constant3/1 -> output3/1
  Constant2/1 -> output2/1
  LCDAL_SEAAlert_Convert/1 -> output1/1
  LCDAL_SEAAlert_L/1 -> LCDAL_SEAAlert_Convert/1
  LCDAL_SEAAlert_Convert1/1 -> LCDAL_SEAAlert_L/1
  LCDAL_SEAAlert_1sat/1 -> LCDAL_SEAAlert_Convert1/1
  LCDAL_SEAAlert_S/1 -> LCDAL_SEAAlert_1sat/1
  LCDAL_SEAAlertRon/1 -> LCDAL_SEAAlert_S/1
  LCDAL_SEAAlert_D/1 -> LCDAL_SEAAlertRon/1
  LCDAL_SEAAlert_F/1 -> LCDAL_SEAAlert_D/2
  LCDAL_SEAAlert_st/1 -> LCDAL_SEAAlert_D/1
  LCDAL_SEAAlert_O/1 -> LCDAL_SEAAlert_st/2
  LCDAL_SEAAlert_sat/1 -> LCDAL_SEAAlert_st/1
  LCDAL_SEAAlert/1 -> LCDAL_SEAAlert_sat/1

== system VCU_CS75_12_27_test/长安CS75底盘程序，20ms一次/Output/Subsystem/TransmitMessages11/GW_LCDAL_2EA/LCDAL_SEAEnableStatus ==
  LCDAL_SEAEnableStatus : Inport
  Constant{1..2,4..8} (7 alike) : Constant  Value=0  OutDataTypeStr=uint8
  LCDAL_SEAEnableStatusRon : Rounding  Operator=round
  LCDAL_SEAEnableStatus_1sat : Saturate  UpperLimit=12  LowerLimit=0
  LCDAL_SEAEnableStatus_Convert : DataTypeConversion  OutDataTypeStr=uint8
  LCDAL_SEAEnableStatus_Convert1 : DataTypeConversion  OutDataTypeStr=uint32
  LCDAL_SEAEnableStatus_D : Product  Inputs=*/
  LCDAL_SEAEnableStatus_F : Constant  OutDataTypeStr=single
  LCDAL_SEAEnableStatus_L : simulink/Logic and Bit Operations/Bitwise Operator  logicop=AND  UseBitMask=on  BitMask=12  BitMaskRealWorld=Stored Integer
  LCDAL_SEAEnableStatus_O : Constant  Value=0  OutDataTypeStr=single
  LCDAL_SEAEnableStatus_S : ArithShift  BitShiftNumber=-2
  LCDAL_SEAEnableStatus_sat : Saturate  UpperLimit=3  LowerLimit=0
  LCDAL_SEAEnableStatus_st : Sum  Inputs=+-
  output1 : Outport
  output2 : Outport  Port=2
  output3 : Outport  Port=3
  output4 : Outport  Port=4
  output5 : Outport  Port=5
  output6 : Outport  Port=6
  output7 : Outport  Port=7
  output8 : Outport  Port=8
  wires:
  Constant8/1 -> output8/1
  Constant7/1 -> output7/1
  Constant6/1 -> output6/1
  Constant5/1 -> output5/1
  Constant4/1 -> output4/1
  Constant2/1 -> output2/1
  Constant1/1 -> output1/1
  LCDAL_SEAEnableStatus_Convert/1 -> output3/1
  LCDAL_SEAEnableStatus_L/1 -> LCDAL_SEAEnableStatus_Convert/1
  LCDAL_SEAEnableStatus_Convert1/1 -> LCDAL_SEAEnableStatus_L/1
  LCDAL_SEAEnableStatus_1sat/1 -> LCDAL_SEAEnableStatus_Convert1/1
  LCDAL_SEAEnableStatus_S/1 -> LCDAL_SEAEnableStatus_1sat/1
  LCDAL_SEAEnableStatusRon/1 -> LCDAL_SEAEnableStatus_S/1
  LCDAL_SEAEnableStatus_D/1 -> LCDAL_SEAEnableStatusRon/1
  LCDAL_SEAEnableStatus_F/1 -> LCDAL_SEAEnableStatus_D/2
  LCDAL_SEAEnableStatus_st/1 -> LCDAL_SEAEnableStatus_D/1
  LCDAL_SEAEnableStatus_O/1 -> LCDAL_SEAEnableStatus_st/2
  LCDAL_SEAEnableStatus_sat/1 -> LCDAL_SEAEnableStatus_st/1
  LCDAL_SEAEnableStatus/1 -> LCDAL_SEAEnableStatus_sat/1

== system VCU_CS75_12_27_test/长安CS75底盘程序，20ms一次/Output/Subsystem/TransmitMessages11/GW_LCDAL_2EA/LCDAL_SEAStatus ==
  LCDAL_SEAStatus : Inport
  Constant{1..2,4..8} (7 alike) : Constant  Value=0  OutDataTypeStr=uint8
  LCDAL_SEAStatusRon : Rounding  Operator=round
  LCDAL_SEAStatus_1sat : Saturate  UpperLimit=192  LowerLimit=0
  LCDAL_SEAStatus_Convert : DataTypeConversion  OutDataTypeStr=uint8
  LCDAL_SEAStatus_Convert1 : DataTypeConversion  OutDataTypeStr=uint32
  LCDAL_SEAStatus_D : Product  Inputs=*/
  LCDAL_SEAStatus_F : Constant  OutDataTypeStr=single
  LCDAL_SEAStatus_L : simulink/Logic and Bit Operations/Bitwise Operator  logicop=AND  UseBitMask=on  BitMask=192  BitMaskRealWorld=Stored Integer
  LCDAL_SEAStatus_O : Constant  Value=0  OutDataTypeStr=single
  LCDAL_SEAStatus_S : ArithShift  BitShiftNumber=-6
  LCDAL_SEAStatus_sat : Saturate  UpperLimit=3  LowerLimit=0
  LCDAL_SEAStatus_st : Sum  Inputs=+-
  output1 : Outport
  output2 : Outport  Port=2
  output3 : Outport  Port=3
  output4 : Outport  Port=4
  output5 : Outport  Port=5
  output6 : Outport  Port=6
  output7 : Outport  Port=7
  output8 : Outport  Port=8
  wires:
  Constant8/1 -> output8/1
  Constant7/1 -> output7/1
  Constant6/1 -> output6/1
  Constant5/1 -> output5/1
  Constant4/1 -> output4/1
  Constant2/1 -> output2/1
  Constant1/1 -> output1/1
  LCDAL_SEAStatus_Convert/1 -> output3/1
  LCDAL_SEAStatus_L/1 -> LCDAL_SEAStatus_Convert/1
  LCDAL_SEAStatus_Convert1/1 -> LCDAL_SEAStatus_L/1
  LCDAL_SEAStatus_1sat/1 -> LCDAL_SEAStatus_Convert1/1
  LCDAL_SEAStatus_S/1 -> LCDAL_SEAStatus_1sat/1
  LCDAL_SEAStatusRon/1 -> LCDAL_SEAStatus_S/1
  LCDAL_SEAStatus_D/1 -> LCDAL_SEAStatusRon/1
  LCDAL_SEAStatus_F/1 -> LCDAL_SEAStatus_D/2
  LCDAL_SEAStatus_st/1 -> LCDAL_SEAStatus_D/1
  LCDAL_SEAStatus_O/1 -> LCDAL_SEAStatus_st/2
  LCDAL_SEAStatus_sat/1 -> LCDAL_SEAStatus_st/1
  LCDAL_SEAStatus/1 -> LCDAL_SEAStatus_sat/1

== system VCU_CS75_12_27_test/长安CS75底盘程序，20ms一次/Output/Subsystem/TransmitMessages11/GW_LCDAL_2EA/LCDAL_SystemStatus ==
  LCDAL_SystemStatus : Inport
  Constant{1,3..8} (7 alike) : Constant  Value=0  OutDataTypeStr=uint8
  LCDAL_SystemStatusRon : Rounding  Operator=round
  LCDAL_SystemStatus_1sat : Saturate  UpperLimit=224  LowerLimit=0
  LCDAL_SystemStatus_Convert : DataTypeConversion  OutDataTypeStr=uint8
  LCDAL_SystemStatus_Convert1 : DataTypeConversion  OutDataTypeStr=uint32
  LCDAL_SystemStatus_D : Product  Inputs=*/
  LCDAL_SystemStatus_F : Constant  OutDataTypeStr=single
  LCDAL_SystemStatus_L : simulink/Logic and Bit Operations/Bitwise Operator  logicop=AND  UseBitMask=on  BitMask=224  BitMaskRealWorld=Stored Integer
  LCDAL_SystemStatus_O : Constant  Value=0  OutDataTypeStr=single
  LCDAL_SystemStatus_S : ArithShift  BitShiftNumber=-5
  LCDAL_SystemStatus_sat : Saturate  UpperLimit=7  LowerLimit=0
  LCDAL_SystemStatus_st : Sum  Inputs=+-
  output1 : Outport
  output2 : Outport  Port=2
  output3 : Outport  Port=3
  output4 : Outport  Port=4
  output5 : Outport  Port=5
  output6 : Outport  Port=6
  output7 : Outport  Port=7
  output8 : Outport  Port=8
  wires:
  Constant8/1 -> output8/1
  Constant7/1 -> output7/1
  Constant6/1 -> output6/1
  Constant5/1 -> output5/1
  Constant4/1 -> output4/1
  Constant3/1 -> output3/1
  Constant1/1 -> output1/1
  LCDAL_SystemStatus_Convert/1 -> output2/1
  LCDAL_SystemStatus_L/1 -> LCDAL_SystemStatus_Convert/1
  LCDAL_SystemStatus_Convert1/1 -> LCDAL_SystemStatus_L/1
  LCDAL_SystemStatus_1sat/1 -> LCDAL_SystemStatus_Convert1/1
  LCDAL_SystemStatus_S/1 -> LCDAL_SystemStatus_1sat/1
  LCDAL_SystemStatusRon/1 -> LCDAL_SystemStatus_S/1
  LCDAL_SystemStatus_D/1 -> LCDAL_SystemStatusRon/1
  LCDAL_SystemStatus_F/1 -> LCDAL_SystemStatus_D/2
  LCDAL_SystemStatus_st/1 -> LCDAL_SystemStatus_D/1
  LCDAL_SystemStatus_O/1 -> LCDAL_SystemStatus_st/2
  LCDAL_SystemStatus_sat/1 -> LCDAL_SystemStatus_st/1
  LCDAL_SystemStatus/1 -> LCDAL_SystemStatus_sat/1

== system VCU_CS75_12_27_test/长安CS75底盘程序，20ms一次/Output/Subsystem/TransmitMessages13/GW_LCDAR_2FA/LCDAR_BSDLCAAlert ==
  LCDAR_BSDLCAAlert : Inport
  Constant{2..8} (7 alike) : Constant  Value=0  OutDataTypeStr=uint8
  LCDAR_BSDLCAAlertRon : Rounding  Operator=round
  LCDAR_BSDLCAAlert_1sat : Saturate  UpperLimit=48  LowerLimit=0
  LCDAR_BSDLCAAlert_Convert : DataTypeConversion  OutDataTypeStr=uint8
  LCDAR_BSDLCAAlert_Convert1 : DataTypeConversion  OutDataTypeStr=uint32
  LCDAR_BSDLCAAlert_D : Product  Inputs=*/
  LCDAR_BSDLCAAlert_F : Constant  OutDataTypeStr=single
  LCDAR_BSDLCAAlert_L : simulink/Logic and Bit Operations/Bitwise Operator  logicop=AND  UseBitMask=on  BitMask=48  BitMaskRealWorld=Stored Integer
  LCDAR_BSDLCAAlert_O : Constant  Value=0  OutDataTypeStr=single
  LCDAR_BSDLCAAlert_S : ArithShift  BitShiftNumber=-4
  LCDAR_BSDLCAAlert_sat : Saturate  UpperLimit=3  LowerLimit=0
  LCDAR_BSDLCAAlert_st : Sum  Inputs=+-
  output1 : Outport
  output2 : Outport  Port=2
  output3 : Outport  Port=3
  output4 : Outport  Port=4
  output5 : Outport  Port=5
  output6 : Outport  Port=6
  output7 : Outport  Port=7
  output8 : Outport  Port=8
  wires:
  LCDAR_BSDLCAAlert/1 -> LCDAR_BSDLCAAlert_sat/1
  LCDAR_BSDLCAAlert_sat/1 -> LCDAR_BSDLCAAlert_st/1
  LCDAR_BSDLCAAlert_O/1 -> LCDAR_BSDLCAAlert_st/2
  LCDAR_BSDLCAAlert_st/1 -> LCDAR_BSDLCAAlert_D/1
  LCDAR_BSDLCAAlert_F/1 -> LCDAR_BSDLCAAlert_D/2
  LCDAR_BSDLCAAlert_D/1 -> LCDAR_BSDLCAAlertRon/1
  LCDAR_BSDLCAAlertRon/1 -> LCDAR_BSDLCAAlert_S/1
  LCDAR_BSDLCAAlert_S/1 -> LCDAR_BSDLCAAlert_1sat/1
  LCDAR_BSDLCAAlert_1sat/1 -> LCDAR_BSDLCAAlert_Convert1/1
  LCDAR_BSDLCAAlert_Convert1/1 -> LCDAR_BSDLCAAlert_L/1
  LCDAR_BSDLCAAlert_L/1 -> LCDAR_BSDLCAAlert_Convert/1
  LCDAR_BSDLCAAlert_Convert/1 -> output1/1
  Constant2/1 -> output2/1
  Constant3/1 -> output3/1
  Constant4/1 -> output4/1
  Constant5/1 -> output5/1
  Constant6/1 -> output6/1
  Constant7/1 -> output7/1
  Constant8/1 -> output8/1

== system VCU_CS75_12_27_test/长安CS75底盘程序，20ms一次/Output/Subsystem/TransmitMessages13/GW_LCDAR_2FA/LCDAR_BSDLCAStatus ==
  LCDAR_BSDLCAStatus : Inport
  Constant{1,3..8} (7 alike) : Constant  Value=0  OutDataTypeStr=uint8
  LCDAR_BSDLCAStatusRon : Rounding  Operator=round
  LCDAR_BSDLCAStatus_1sat : Saturate  UpperLimit=24  LowerLimit=0
  LCDAR_BSDLCAStatus_Convert : DataTypeConversion  OutDataTypeStr=uint8
  LCDAR_BSDLCAStatus_Convert1 : DataTypeConversion  OutDataTypeStr=uint32
  LCDAR_BSDLCAStatus_D : Product  Inputs=*/
  LCDAR_BSDLCAStatus_F : Constant  OutDataTypeStr=single
  LCDAR_BSDLCAStatus_L : simulink/Logic and Bit Operations/Bitwise Operator  logicop=AND  UseBitMask=on  BitMask=24  BitMaskRealWorld=Stored Integer
  LCDAR_BSDLCAStatus_O : Constant  Value=0  OutDataTypeStr=single
  LCDAR_BSDLCAStatus_S : ArithShift  BitShiftNumber=-3
  LCDAR_BSDLCAStatus_sat : Saturate  UpperLimit=3  LowerLimit=0
  LCDAR_BSDLCAStatus_st : Sum  Inputs=+-
  output1 : Outport
  output2 : Outport  Port=2
  output3 : Outport  Port=3
  output4 : Outport  Port=4
  output5 : Outport  Port=5
  output6 : Outport  Port=6
  output7 : Outport  Port=7
  output8 : Outport  Port=8
  wires:
  LCDAR_BSDLCAStatus/1 -> LCDAR_BSDLCAStatus_sat/1
  LCDAR_BSDLCAStatus_sat/1 -> LCDAR_BSDLCAStatus_st/1
  LCDAR_BSDLCAStatus_O/1 -> LCDAR_BSDLCAStatus_st/2
  LCDAR_BSDLCAStatus_st/1 -> LCDAR_BSDLCAStatus_D/1
  LCDAR_BSDLCAStatus_F/1 -> LCDAR_BSDLCAStatus_D/2
  LCDAR_BSDLCAStatus_D/1 -> LCDAR_BSDLCAStatusRon/1
  LCDAR_BSDLCAStatusRon/1 -> LCDAR_BSDLCAStatus_S/1
  LCDAR_BSDLCAStatus_S/1 -> LCDAR_BSDLCAStatus_1sat/1
  LCDAR_BSDLCAStatus_1sat/1 -> LCDAR_BSDLCAStatus_Convert1/1
  LCDAR_BSDLCAStatus_Convert1/1 -> LCDAR_BSDLCAStatus_L/1
  LCDAR_BSDLCAStatus_L/1 -> LCDAR_BSDLCAStatus_Convert/1
  LCDAR_BSDLCAStatus_Convert/1 -> output2/1
  Constant1/1 -> output1/1
  Constant3/1 -> output3/1
  Constant4/1 -> output4/1
  Constant5/1 -> output5/1
  Constant6/1 -> output6/1
  Constant7/1 -> output7/1
  Constant8/1 -> output8/1

== system VCU_CS75_12_27_test/长安CS75底盘程序，20ms一次/Output/Subsystem/TransmitMessages13/GW_LCDAR_2FA/LCDAR_CTAAlert ==
  LCDAR_CTAAlert : Inport
  Constant{2..8} (7 alike) : Constant  Value=0  OutDataTypeStr=uint8
  LCDAR_CTAAlertABS : Abs
  LCDAR_CTAAlertCS : ArithShift  BitShiftNumber=-2
  LCDAR_CTAAlertConS : Constant  OutDataTypeStr=single
  LCDAR_CTAAlertCosR : Constant  Value=0  OutDataTypeStr=uint8
  LCDAR_CTAAlertROP : RelationalOperator  Operator=<  OutDataTypeStr=boolean
  LCDAR_CTAAlertRon : Rounding  Operator=round
  LCDAR_CTAAlertSW : Switch  Criteria=u2 ~= 0
  LCDAR_CTAAlert_1sat : Saturate  UpperLimit=3  LowerLimit=0
  LCDAR_CTAAlert_Convert : DataTypeConversion  OutDataTypeStr=uint8
  LCDAR_CTAAlert_Convert1 : DataTypeConversion  OutDataTypeStr=uint32
  LCDAR_CTAAlert_D : Product  Inputs=*/
  LCDAR_CTAAlert_F : Constant  OutDataTypeStr=single
  LCDAR_CTAAlert_L : simulink/Logic and Bit Operations/Bitwise Operator  logicop=AND  UseBitMask=on  BitMask=3  BitMaskRealWorld=Stored Integer
  LCDAR_CTAAlert_O : Constant  Value=0  OutDataTypeStr=single
  LCDAR_CTAAlert_S : ArithShift
  LCDAR_CTAAlert_sat : Saturate  UpperLimit=3  LowerLimit=0
  LCDAR_CTAAlert_st : Sum  Inputs=+-
  LCDAR_CTAAlertsubcon : Sum  Inputs=+-
  output1 : Outport
  output2 : Outport  Port=2
  output3 : Outport  Port=3
  output4 : Outport  Port=4
  output5 : Outport  Port=5
  output6 : Outport  Port=6
  output7 : Outport  Port=7
  output8 : Outport  Port=8
  wires:
  LCDAR_CTAAlert/1 -> LCDAR_CTAAlert_sat/1
  LCDAR_CTAAlert_sat/1 -> LCDAR_CTAAlert_st/1
  LCDAR_CTAAlert_O/1 -> LCDAR_CTAAlert_st/2
  LCDAR_CTAAlert_st/1 -> LCDAR_CTAAlert_D/1
  LCDAR_CTAAlert_F/1 -> LCDAR_CTAAlert_D/2
  LCDAR_CTAAlert_D/1 -> LCDAR_CTAAlertRon/1
  LCDAR_CTAAlertRon/1 -> LCDAR_CTAAlertROP/1, LCDAR_CTAAlertABS/1, LCDAR_CTAAlertSW/3
  LCDAR_CTAAlertCosR/1 -> LCDAR_CTAAlertROP/2
  LCDAR_CTAAlertConS/1 -> LCDAR_CTAAlertCS/1
  LCDAR_CTAAlertCS/1 -> LCDAR_CTAAlertsubcon/1
  LCDAR_CTAAlertABS/1 -> LCDAR_CTAAlertsubcon/2
  LCDAR_CTAAlertsubcon/1 -> LCDAR_CTAAlertSW/1
  LCDAR_CTAAlertROP/1 -> LCDAR_CTAAlertSW/2
  LCDAR_CTAAlertSW/1 -> LCDAR_CTAAlert_S/1
  LCDAR_CTAAlert_S/1 -> LCDAR_CTAAlert_1sat/1
  LCDAR_CTAAlert_1sat/1 -> LCDAR_CTAAlert_Convert1/1
  LCDAR_CTAAlert_Convert1/1 -> LCDAR_CTAAlert_L/1
  LCDAR_CTAAlert_L/1 -> LCDAR_CTAAlert_Convert/1
  LCDAR_CTAAlert_Convert/1 -> output1/1
  Constant2/1 -> output2/1
  Constant3/1 -> output3/1
  Constant4/1 -> output4/1
  Constant5/1 -> output5/1
  Constant6/1 -> output6/1
  Constant7/1 -> output7/1
  Constant8/1 -> output8/1
